simulink model "Motor_Simulation2"  (R2025b)
settings: Solver=FixedStepAuto  StartTime=0.0  StopTime=inf  FixedStep=0.0001  RelTol=1e-3  EnableMultiTasking=on
libraries: raspberrypiNetworklib x1
settings Model: SimulationMode=external  ExtModeTrigDuration=2  Creator=jujma  LastModifiedBy=jujma
settings SolverCC: PositivePriorityOrder=on  AutoInsertRateTranBlk=on
settings OptimizationCC: EnhancedBackFolding=on  PassReuseOutputArgsAs=Individual arguments  ZeroExternalMemoryAtStartup=off  ZeroInternalMemoryAtStartup=off  MaxStackSize=200000  OptimizeBlockOrder=speed  DifferentSizesBufferReuse=on  OptimizationCustomize=off  EfficientTunableParamExpr=on
settings DebuggingCC: ParameterTunabilityLossMsg=error
settings HardwareCC: ProdBitPerPointer=32.0  ProdBitPerSizeT=32.0  ProdBitPerPtrDiffT=32.0  ProdLargestAtomicInteger=Long  ProdLargestAtomicFloat=Double  ProdWordSize=32.0  ProdLongLongMode=on  ProdHWDeviceType=ARM Compatible->ARM Cortex-A (32-bit)
settings RTWCC: SystemTargetFile=ert.tlc  HardwareBoard=Raspberry Pi  TLCOptions="-aInlineSetEventsForThisBaseRateFcn=TLC_FALSE -aSuppressMultiTaskScheduler=TLC_FALSE  -aRateBasedStepFcn=0"  TemplateMakefile=ert_default_tmf  Toolchain=GNU GCC Embedded Linux  BuildConfiguration=Faster Runs  Description=Embedded Coder
settings CodeAppCC: ForceParamTrailComments=on  IgnoreCustomStorageClasses=off  OperatorAnnotations=on  SimulinkDataObjDesc=on  SFDataObjDesc=on  InsertBlockDesc=on
settings ERTTargetCC: ExtModeTransport=2.0  ExtModeStaticAlloc=on  ExtModeMexFile=ext_xcp  ExtModeIntrfLevel=Level2 - Open  InlinedParameterPlacement=Hierarchical  CodeReplacementLibrary=ARM Cortex-A CMSIS  SupportContinuousTime=on  SupportVariableSizeSignals=on

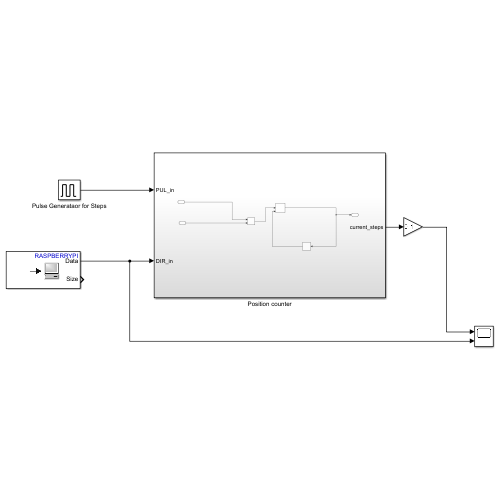
[thumbnail: Simulink's stored preview of the top-level diagram]
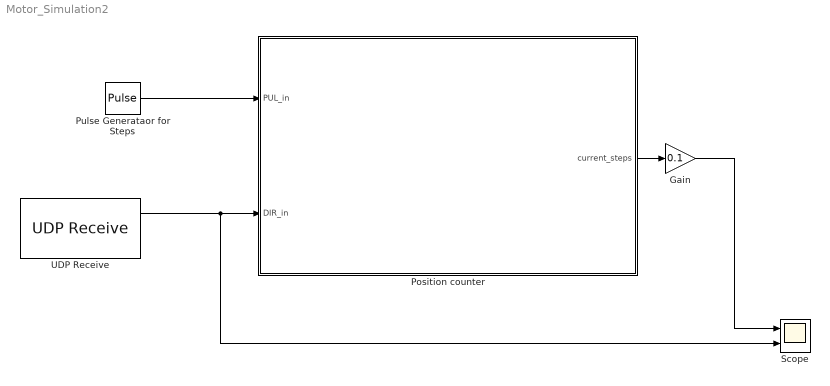
== system Motor_Simulation2 ==
  Gain : Gain  Gain=0.1
  Position counter : Subsystem
  Pulse Generataor for Steps : DiscretePulseGenerator  PulseType=Time based  Period=0.01  PulseWidth=50
  Scope : Scope  NumInputPorts=2
      settings: ActiveDisplayYMinimum=-292.94999999999993  ActiveDisplayYMaximum=2636.5499999999997
  UDP Receive : raspberrypiNetworklib/UDP Receive  localURL='0.0.0.0'  localPort=55001  remoteURL='0.0.0.0'  remotePort=-1  recvBufferSize=8192  signalDatatype=double  dims=2  isVarSize=off  showBlockingTime=off  blockingTime=0  sampletime=0.0001  blockPlatform=Raspberry Pi
  wires:
  Position counter/1(current_steps) -> Gain/1
  UDP Receive/1 -> Scope/2, Position counter/2(DIR_in)
  Pulse Generataor for Steps/1 -> Position counter/1(PUL_in)
  Gain/1 -> Scope/1

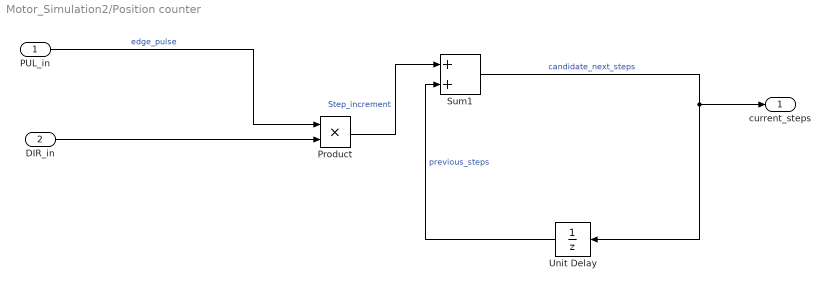
== system Motor_Simulation2/Position counter ==
  PUL_in : Inport
  DIR_in : Inport  Port=2
  Product : Product
  Sum1 : Sum  Inputs=|++
  Unit Delay : UnitDelay  SampleTime=0.0001  HasFrameUpgradeWarning=on
  current_steps : Outport
  wires:
  PUL_in/1 -> Product/1  "edge_pulse"
  DIR_in/1 -> Product/2
  Product/1 -> Sum1/1  "Step_increment"
  Unit Delay/1 -> Sum1/2  "previous_steps"
  Sum1/1 -> Unit Delay/1, current_steps/1  "candidate_next_steps"
